simulink model "Grading_System"  (R2021a)
settings: Solver=FixedStepDiscrete  StartTime=0.0  StopTime=10.0  RelTol=1e-3  EnableMultiTasking=on
settings Model: Creator=Osman  LastModifiedBy=Osman
settings DataIOCC: ReturnWorkspaceOutputs=off
settings OptimizationCC: DefaultParameterBehavior=Inlined  InlineInvariantSignals=on  EnableMemcpy=off  LifeSpan=1  EfficientTunableParamExpr=on
settings DebuggingCC: UnderspecifiedInitializationDetection=Classic  MergeDetectMultiDrivingBlocksExec=none  SFMachineParentedDataDiag=warning  ArithmeticOperatorsInVariantConditions=warning
settings ModelReferenceCC: PropagateSignalLabelsOutOfModel=off
settings SFSimCC: MATLABDynamicMemAlloc=off  CustomCodeUndefinedFunction=UseInterfaceOnly
settings RTWCC: SystemTargetFile=ert.tlc  GenCodeOnly=on  TemplateMakefile=ert_default_tmf  GenerateReport=on  IncludeHyperlinkInReport=on  LaunchReport=on  GenerateTraceInfo=on  GenerateTraceReport=on  GenerateTraceReportSl=on  GenerateTraceReportSf=on  GenerateTraceReportEml=on
settings CodeAppCC: ForceParamTrailComments=on  IgnoreCustomStorageClasses=off  OperatorAnnotations=on  SimulinkDataObjDesc=on  SFDataObjDesc=on  MATLABFcnDesc=on  InsertBlockDesc=on  StateflowObjectComments=on  MATLABSourceComments=on
settings ERTTargetCC: MultiwordLength=2048  GenerateSampleERTMain=on  InlinedParameterPlacement=NonHierarchical  ERTCustomFileTemplate=example_file_process.tlc

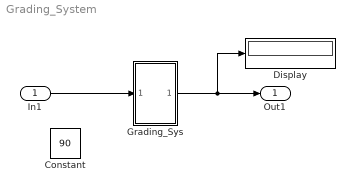
== system Grading_System ==
  In1 : Inport
  Constant : Constant  Value=90
  Display : Display
  Grading_Sys : Subsystem
  Out1 : Outport
  wires:
  Grading_Sys/1(Out1) -> Display/1, Out1/1
  In1/1 -> Grading_Sys/1(In1)

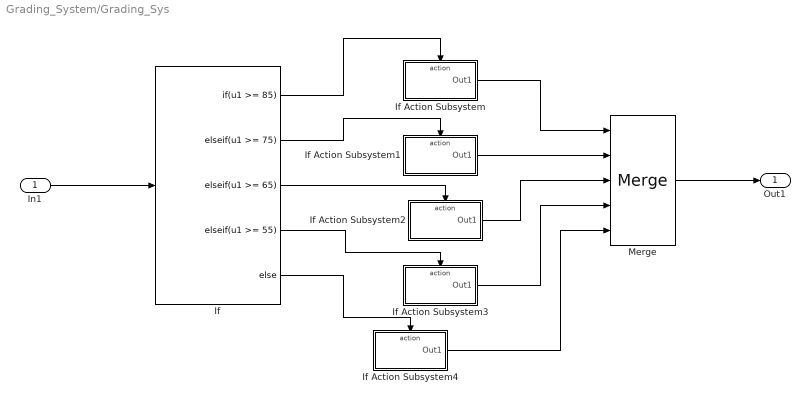
== system Grading_System/Grading_Sys ==
  In1 : Inport
  If : If  IfExpression=u1 >= 85  ElseIfExpressions=u1 >= 75, u1 >= 65, u1 >= 55
  If Action Subsystem : Subsystem  TreatAsAtomicUnit=on
  If Action Subsystem1 : Subsystem  TreatAsAtomicUnit=on
  If Action Subsystem2 : Subsystem  TreatAsAtomicUnit=on
  If Action Subsystem3 : Subsystem  TreatAsAtomicUnit=on
  If Action Subsystem4 : Subsystem  TreatAsAtomicUnit=on
  Merge : Merge  Inputs=5
  Out1 : Outport
  wires:
  If/4 -> If Action Subsystem3/Action
  If Action Subsystem4/1(Out1) -> Merge/5
  If/3 -> If Action Subsystem2/Action
  If/1 -> If Action Subsystem/Action
  If Action Subsystem2/1(Out1) -> Merge/3
  If/5 -> If Action Subsystem4/Action
  Merge/1 -> Out1/1
  If/2 -> If Action Subsystem1/Action
  If Action Subsystem1/1(Out1) -> Merge/2
  If Action Subsystem3/1(Out1) -> Merge/4
  If Action Subsystem/1(Out1) -> Merge/1
  In1/1 -> If/1

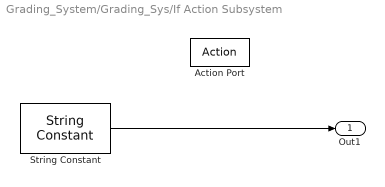
== system Grading_System/Grading_Sys/If Action Subsystem ==
  Action Port : ActionPort  ActionPortLabel=if(u1 >= 85)
  String Constant : StringConstant  String="\"A\""
  Out1 : Outport
  wires:
  String Constant/1 -> Out1/1

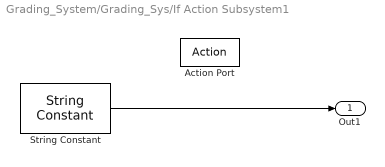
== system Grading_System/Grading_Sys/If Action Subsystem1 ==
  Action Port : ActionPort  ActionPortLabel=elseif(u1 >= 75)
  String Constant : StringConstant  String="\"B\""
  Out1 : Outport
  wires:
  String Constant/1 -> Out1/1

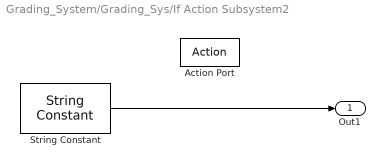
== system Grading_System/Grading_Sys/If Action Subsystem2 ==
  Action Port : ActionPort  ActionPortLabel=elseif( u1 >= 65)
  String Constant : StringConstant  String="\"C\""
  Out1 : Outport
  wires:
  String Constant/1 -> Out1/1

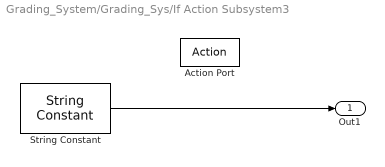
== system Grading_System/Grading_Sys/If Action Subsystem3 ==
  Action Port : ActionPort  ActionPortLabel=elseif( u1 >= 55)
  String Constant : StringConstant  String="\"D\""
  Out1 : Outport
  wires:
  String Constant/1 -> Out1/1

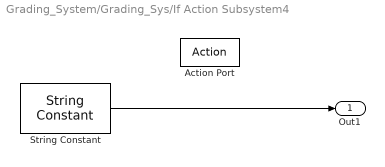
== system Grading_System/Grading_Sys/If Action Subsystem4 ==
  Action Port : ActionPort  ActionPortLabel=else
  String Constant : StringConstant  String="\"F\""
  Out1 : Outport
  wires:
  String Constant/1 -> Out1/1
